simulink model "Control_dron"  (R2025a)
settings: Solver=VariableStepAuto  StartTime=0.0  StopTime=20  RelTol=1e-3
libraries: slpidlib x1
settings Model: Creator=minez  LastModifiedBy=minez

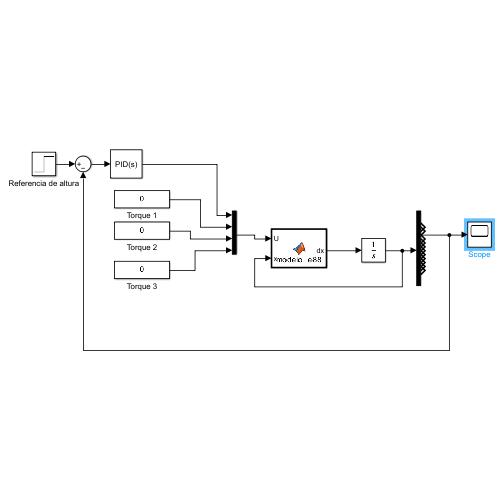
[thumbnail: Simulink's stored preview of the top-level diagram]
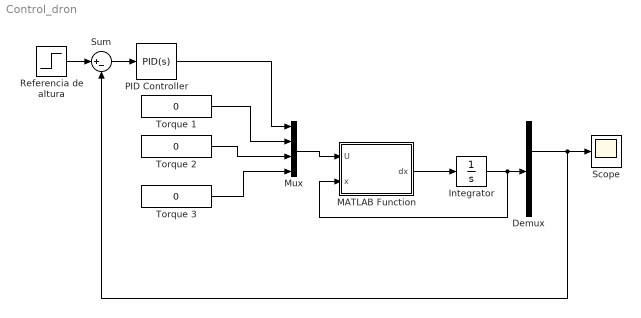
== system Control_dron ==
  Demux : Demux  Outputs=12
  Integrator : Integrator  InitialCondition=zeros(12,1)
  MATLAB Function : MATLAB Function  TreatAsAtomicUnit=on
  Mux : Mux
  PID Controller : slpidlib/PID Controller  Controller=PID  Form=Parallel  TimeDomain=Continuous-time  UseExternalTs=off  SampleTime=-1  IntegratorMethod=Forward Euler  FilterMethod=Forward Euler  ControllerParametersSource=internal  P=10  I=10  UseKiTs=off  D=9  UseExternalDerivativeSource=off  N=20  UseFilter=on  TunerSelectOption=Transfer Function Based (PID Tuner App)  InitialConditionSource=internal  InitialConditionForIntegrator=0  InitialConditionForFilter=0  DifferentiatorICPrevScaledInput=0  ExternalReset=none  TrackingMode=off  Kt=1  LimitOutput=off  SatLimitsSource=internal  UpperSaturationLimit=6  LowerSaturationLimit=0  LinearizeAsGain=on  AntiWindupMode=none  Kb=1  LimitIntegrator=off  UpperIntegratorSaturationLimit=inf  LowerIntegratorSaturationLimit=-inf  POutMin=[]  POutMax=[]  IOutMin=[]  IOutMax=[]  DOutMin=[]  DOutMax=[]  NOutMin=[]  NOutMax=[]  SumOutMin=[]  SumOutMax=[]  SaturationOutMin=[]  SaturationOutMax=[]  PParamMin=[]  PParamMax=[]  IParamMin=[]  IParamMax=[]  DParamMin=[]  DParamMax=[]  NParamMin=[]  NParamMax=[]  KbParamMin=[]  KbParamMax=[]  KtParamMin=[]  KtParamMax=[]  KbOutMin=[]  KbOutMax=[]  KtOutMin=[]  KtOutMax=[]  IntegratorOutMin=[]  IntegratorOutMax=[]  FilterOutMin=[]  FilterOutMax=[]  SumI1OutMin=[]  SumI1OutMax=[]  SumI2OutMin=[]  SumI2OutMax=[]  SumI3OutMin=[]  SumI3OutMax=[]  SumI4OutMin=[]  SumI4OutMax=[]  SumDOutMin=[]  SumDOutMax=[]  DifferentiatorOutMin=[]  DifferentiatorOutMax=[]  FilterDiffOutCoefMin=[]  FilterDiffOutCoefMax=[]  ReciprocalOutMin=[]  ReciprocalOutMax=[]  SumDenOutMin=[]  SumDenOutMax=[]  SumNumOutMin=[]  SumNumOutMax=[]  DivideOutMin=[]  DivideOutMax=[]  UdiffTsProdOutMin=[]  UdiffTsProdOutMax=[]  NTsProdOutMin=[]  NTsProdOutMax=[]  UintegralTsProdOutMin=[]  UintegralTsProdOutMax=[]  UngainTsProdOutMin=[]  UngainTsProdOutMax=[]  ClampingZeroOutDataTypeStr=Inherit: Inherit via back propagation  ClampingZeroOutMin=[]  ClampingZeroOutMax=[]  FilterDenConstantOutDataTypeStr=Inherit: Inherit via back propagation  FilterDenConstantOutMin=[]  FilterDenConstantOutMax=[]  PCopyOutDataTypeStr=Inherit: Inherit via back propagation  PCopyOutMin=[]  PCopyOutMax=[]  NCopyOutDataTypeStr=Inherit: Inherit via back propagation  NCopyOutMin=[]  NCopyOutMax=[]  IntegratorContinuousStateAttributes=''  IntegratorStateMustResolveToSignalObject=off  IntegratorRTWStateStorageClass=Auto  FilterContinuousStateAttributes=''  FilterStateMustResolveToSignalObject=off  FilterRTWStateStorageClass=Auto  ParallelPVariant=InternalParameters  IdealPVariant=Disabled  IVariant=InternalParameters  DVariant=InternalParameters  IntegratorVariant=Continuous  SatVariant=Disabled  AWVariant=Passthrough  PCopyVariant=Disabled  TRVariant=Disabled  FdbkBlocksVariant=Forward  IdealPFdbkVariant=Disabled  SatFdbkVariant=Disabled  DerivativeFilterVariant=ContFilter  NVariant=InternalParameters  NCopyVariant=Disabled  FilterICVariant=InternalICsFilter  IntegratorICVariant=InternalICs  ExternalResetVariant=Disabled  TRSumVariant=Passthrough  SumFdbkVariant=Disabled  SumVariant=Sum_PID  TsampFilterVariant=InternalTs  TsampNgainVariant=Passthrough  TsampIntegralVariant=Disabled_SignalSpec  ExternalSaturationOutDataTypeStr=Inherit: Same as second input  DerivativeSourceVariant=ErrorSignal  PreIntVariant=InternalPreInt
  Referencia de altura : Step  After=2  SampleTime=0
  Scope : Scope
      settings: ActiveDisplayYMinimum=-2.1239296000172541  ActiveDisplayYMaximum=4.2922383558455222
  Sum : Sum  Inputs=|+-
  Torque 1 : Constant  Value=0
  Torque 2 : Constant  Value=0
  Torque 3 : Constant  Value=0
  wires:
  MATLAB Function/1(dx) -> Integrator/1
  Integrator/1 -> MATLAB Function/2(x), Demux/1
  Torque 3/1 -> Mux/4
  Torque 2/1 -> Mux/3
  Torque 1/1 -> Mux/2
  Mux/1 -> MATLAB Function/1(U)
  Sum/1 -> PID Controller/1
  Referencia de altura/1 -> Sum/1
  Demux/3 -> Sum/2, Scope/1
  PID Controller/1 -> Mux/1

== matlab function Control_dron/MATLAB Function ==
  data: U input; dx output; x input
function dx = modelo_e88(U, x)
    % Entradas del bloque:
    % U = Vector de 4 posiciones [U1; U2; U3; U4] -> Empuje y Torques
    % x = Vector de estado de 12 posiciones (Posición, ángulos y velocidades)

    % 1. Parámetros Físicos (Valores base del E88, ¡cámbialos por los tuyos luego!)
    m = 0.480;      % Masa total en kg (80 gramos)
    g = 9.81;       % Gravedad en m/s^2
    Ixx = 4.0e-4;   % Inercia en X (Aproximación)
    Iyy = 4.0e-4;   % Inercia en Y (Aproximación)
    Izz = 8.0e-4;   % Inercia en Z (Aproximación)

    % 2. Extracción de los estados actuales del vector 'x'
    % x(1), x(2), x(3) son X, Y, Z (No se usan en la derivada, pero existen)
    
    phi   = x(4);   % Roll (Alabeo)
    theta = x(5);   % Pitch (Cabeceo)
    psi   = x(6);   % Yaw (Guiñada)
    
    dX = x(7);      % Velocidad en X
    dY = x(8);      % Velocidad en Y
    dZ = x(9);      % Velocidad en Z
    
    p = x(10);      % Velocidad angular en X
    q = x(11);      % Velocidad angular en Y
    r = x(12);      % Velocidad angular en Z

    % 3. Extracción de las señales de control de los motores
    U1 = U(1); % Fuerza de empuje total (Throttle)
    U2 = U(2); % Torque en Roll
    U3 = U(3); % Torque en Pitch
    U4 = U(4); % Torque en Yaw

    % 4. DINÁMICA DE TRASLACIÓN (Aceleraciones lineales ddX, ddY, ddZ)
    ddX = (U1 / m) * (cos(phi)*sin(theta)*cos(psi) + sin(phi)*sin(psi));
    ddY = (U1 / m) * (cos(phi)*sin(theta)*sin(psi) - sin(phi)*cos(psi));
    ddZ = (U1 / m) * (cos(phi)*cos(theta)) - g;

    % 5. DINÁMICA DE ROTACIÓN (Aceleraciones angulares dp, dq, dr)
    dp = (U2 / Ixx) + ((Iyy - Izz) / Ixx) * q * r;
    dq = (U3 / Iyy) + ((Izz - Ixx) / Iyy) * p * r;
    dr = (U4 / Izz) + ((Ixx - Iyy) / Izz) * p * q;

    % Simplificación para ángulos pequeños: la derivada del ángulo es la velocidad angular
    dphi = p;
    dtheta = q;
    dpsi = r;

    % 6. Armado del vector de salida (Derivadas del estado: dx)
    dx = [dX; dY; dZ; dphi; dtheta; dpsi; ddX; ddY; ddZ; dp; dq; dr];
end
